simulink model "overflowtank_v000"  (R2019b)
settings: Solver=ode4  StartTime=0.0  StopTime=10000  FixedStep=1  RelTol=1e-3
libraries: simulink x5
settings Model: PauseTimes=120  Creator=engineer  LastModifiedBy=engineer

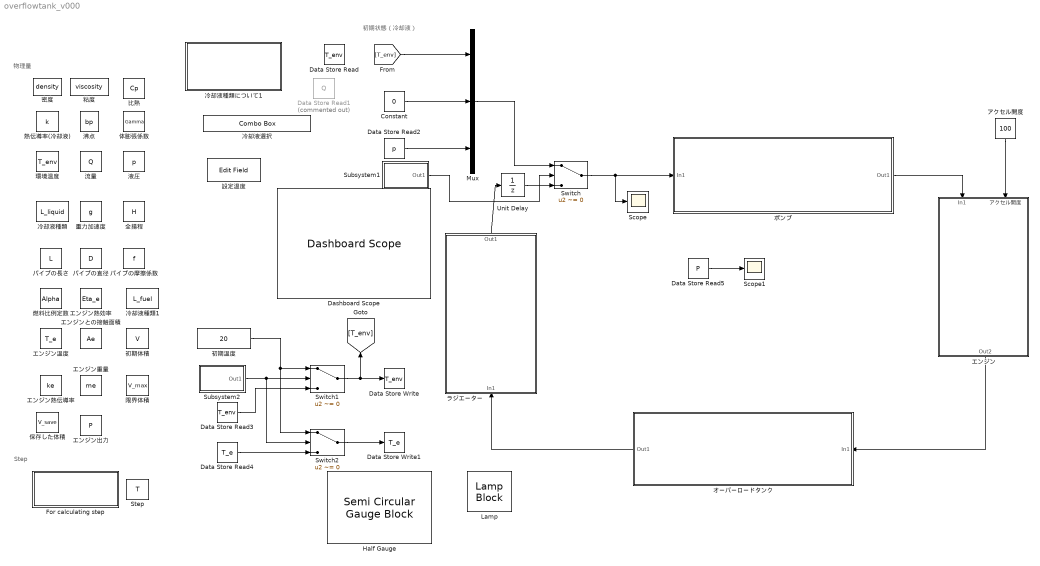
== system overflowtank_v000 ==
  note: 初期状態（冷却液）
  note: 物理量
  note: Step
  " エンジン温度" : DataStoreMemory  DataStoreName=T_e  ReadBeforeWriteMsg=warning  WriteAfterWriteMsg=warning  WriteAfterReadMsg=warning  InitialValue=25  ShowAdditionalParam=off
  " 全揚程" : DataStoreMemory  DataStoreName=H  ReadBeforeWriteMsg=warning  WriteAfterWriteMsg=warning  WriteAfterReadMsg=warning  InitialValue=2  ShowAdditionalParam=off
  " 冷却液種類" : DataStoreMemory  DataStoreName=L_liquid  ReadBeforeWriteMsg=warning  WriteAfterWriteMsg=warning  WriteAfterReadMsg=warning  ShowAdditionalParam=off  OutMin=0  OutMax=2
  " 冷却液種類1" : DataStoreMemory  DataStoreName=L_fuel  ReadBeforeWriteMsg=warning  WriteAfterWriteMsg=warning  WriteAfterReadMsg=warning  ShowAdditionalParam=off  OutMin=0  OutMax=2
  " 流量" : DataStoreMemory  DataStoreName=Q  ReadBeforeWriteMsg=warning  WriteAfterWriteMsg=warning  WriteAfterReadMsg=warning  ShowAdditionalParam=off
  " 液圧" : DataStoreMemory  DataStoreName=p  ReadBeforeWriteMsg=warning  WriteAfterWriteMsg=warning  WriteAfterReadMsg=warning  InitialValue=101  ShowAdditionalParam=off
  " 重力加速度" : DataStoreMemory  DataStoreName=g  ReadBeforeWriteMsg=warning  WriteAfterWriteMsg=warning  WriteAfterReadMsg=warning  InitialValue=10  ShowAdditionalParam=off
  Constant : Constant  Value=0
  Dashboard Scope : DashboardScope
  Data Store Read : DataStoreRead  DataStoreName=T_env
  Data Store Read1 : DataStoreRead  Commented=on  DataStoreName=Q
  Data Store Read2 : DataStoreRead  DataStoreName=p
  Data Store Read3 : DataStoreRead  DataStoreName=T_env
  Data Store Read4 : DataStoreRead  DataStoreName=T_e
  Data Store Read5 : DataStoreRead  DataStoreName=P
  Data Store Write : DataStoreWrite  DataStoreName=T_env
  Data Store Write1 : DataStoreWrite  DataStoreName=T_e
  For calculating step : Subsystem
  Half Gauge : SemiCircularGaugeBlock  ScaleMax=50
  Lamp : LampBlock
  Mux : Mux  Inputs=3
  Scope : Scope
  Scope1 : Scope
  Step : DataStoreMemory  DataStoreName=T  ReadBeforeWriteMsg=warning  WriteAfterWriteMsg=warning  WriteAfterReadMsg=warning  ShowAdditionalParam=off
  Subsystem1 : Subsystem
  Subsystem2 : Subsystem
  Switch : Switch  Criteria=u2 ~= 0
  Switch1 : Switch  Criteria=u2 ~= 0
  Switch2 : Switch  Criteria=u2 ~= 0
  Unit Delay : UnitDelay  SampleTime=-1  HasFrameUpgradeWarning=on
  アクセル開度 : Constant  Value=100
  エンジン : Subsystem
  エンジンとの接触面積 : DataStoreMemory  DataStoreName=Ae  ReadBeforeWriteMsg=warning  WriteAfterWriteMsg=warning  WriteAfterReadMsg=warning  InitialValue=0.3  ShowAdditionalParam=off
  エンジン出力 : DataStoreMemory  DataStoreName=P  ReadBeforeWriteMsg=warning  WriteAfterWriteMsg=warning  WriteAfterReadMsg=warning  ShowAdditionalParam=off
  エンジン熱伝導率 : DataStoreMemory  DataStoreName=ke  ReadBeforeWriteMsg=warning  WriteAfterWriteMsg=warning  WriteAfterReadMsg=warning  InitialValue=237  ShowAdditionalParam=off
  エンジン熱効率 : DataStoreMemory  DataStoreName=Eta_e  ReadBeforeWriteMsg=warning  WriteAfterWriteMsg=warning  WriteAfterReadMsg=warning  InitialValue=0.1  ShowAdditionalParam=off
  エンジン重量 : DataStoreMemory  DataStoreName=me  ReadBeforeWriteMsg=warning  WriteAfterWriteMsg=warning  WriteAfterReadMsg=warning  InitialValue=550  ShowAdditionalParam=off
  オーバーロードタンク : Subsystem
  パイプの摩擦係数 : DataStoreMemory  DataStoreName=f  ReadBeforeWriteMsg=warning  WriteAfterWriteMsg=warning  WriteAfterReadMsg=warning  InitialValue=0.01  ShowAdditionalParam=off
  パイプの直径 : DataStoreMemory  DataStoreName=D  ReadBeforeWriteMsg=warning  WriteAfterWriteMsg=warning  WriteAfterReadMsg=warning  InitialValue=0.04  ShowAdditionalParam=off
  パイプの長さ : DataStoreMemory  DataStoreName=L  ReadBeforeWriteMsg=warning  WriteAfterWriteMsg=warning  WriteAfterReadMsg=warning  InitialValue=7  ShowAdditionalParam=off
  ポンプ : Subsystem
  ラジエーター : Subsystem
  体膨張係数 : DataStoreMemory  DataStoreName=Gamma  ReadBeforeWriteMsg=warning  WriteAfterWriteMsg=warning  WriteAfterReadMsg=warning  InitialValue=0.00021  ShowAdditionalParam=off
  保存した体積 : DataStoreMemory  DataStoreName=V_save  InitialValue=0.001  ShowAdditionalParam=off
  冷却液種類について1 : Subsystem  VariantControl=Variant1
  冷却液選択 : ComboBox  LabelPosition=Hide  SelectedLabel=Water
      settings: Values={{'Water', 'EG30%', 'EG50%'}, [0 1 2]}
  初期体積 : DataStoreMemory  DataStoreName=V  InitialValue=0.009  ShowAdditionalParam=off
  初期温度 : Constant  Value=20
  密度 : DataStoreMemory  DataStoreName=density  ReadBeforeWriteMsg=warning  WriteAfterWriteMsg=warning  WriteAfterReadMsg=warning  InitialValue=1000  ShowAdditionalParam=off
  比熱 : DataStoreMemory  DataStoreName=Cp  ReadBeforeWriteMsg=warning  WriteAfterWriteMsg=warning  WriteAfterReadMsg=warning  InitialValue=4184  ShowAdditionalParam=off
  沸点 : DataStoreMemory  DataStoreName=bp  ReadBeforeWriteMsg=warning  WriteAfterWriteMsg=warning  WriteAfterReadMsg=warning  InitialValue=100  ShowAdditionalParam=off
  熱伝導率(冷却液) : DataStoreMemory  DataStoreName=k  ReadBeforeWriteMsg=warning  WriteAfterWriteMsg=warning  WriteAfterReadMsg=warning  InitialValue=0.606  ShowAdditionalParam=off
  燃料比例定数 : DataStoreMemory  DataStoreName=Alpha  ReadBeforeWriteMsg=warning  WriteAfterWriteMsg=warning  WriteAfterReadMsg=warning  InitialValue=0.005  ShowAdditionalParam=off
  "環境温度 " : DataStoreMemory  DataStoreName=T_env  ReadBeforeWriteMsg=warning  WriteAfterWriteMsg=warning  WriteAfterReadMsg=warning  InitialValue=25  ShowAdditionalParam=off
  粘度 : DataStoreMemory  DataStoreName=viscosity  ReadBeforeWriteMsg=warning  WriteAfterWriteMsg=warning  WriteAfterReadMsg=warning  InitialValue=0.001  ShowAdditionalParam=off
  設定温度 : EditField  LabelPosition=Hide  ShowInitialText=on  Alignment=Center
  限界体積 : DataStoreMemory  DataStoreName=V_max  InitialValue=0.009  ShowAdditionalParam=off
  wires:
  Mux/1 -> Switch/1
  [T_env] -> Mux/1
  Constant/1 -> Mux/2
  Data Store Read2/1 -> Mux/3
  Switch/1 -> ポンプ/1(In1), Scope/1
  オーバーロードタンク/1(Out1) -> ラジエーター/1(In1)
  Subsystem1/1(Out1) -> Switch/2
  Unit Delay/1 -> Switch/3
  アクセル開度/1 -> エンジン/2(アクセル開度)
  ポンプ/1(Out1) -> エンジン/1(In1)
  エンジン/1(Out2) -> オーバーロードタンク/1(In1)
  ラジエーター/1(Out1) -> Unit Delay/1
  初期温度/1 -> Switch1/1, Switch2/1
  Subsystem2/1(Out1) -> Switch2/2, Switch1/2
  Switch1/1 -> Data Store Write/1, [T_env]
  Switch2/1 -> Data Store Write1/1
  Data Store Read3/1 -> Switch1/3
  Data Store Read4/1 -> Switch2/3
  Data Store Read5/1 -> Scope1/1

== system overflowtank_v000/For calculating step ==
  Add1 : Sum  Inputs=+-
  Clock1 : Clock
  Data Store Write : DataStoreWrite  DataStoreName=T
  Unit Delay2 : UnitDelay  SampleTime=-1  HasFrameUpgradeWarning=on
  wires:
  Clock1/1 -> Add1/1, Unit Delay2/1
  Add1/1 -> Data Store Write/1
  Unit Delay2/1 -> Add1/2

== system overflowtank_v000/Subsystem1 ==
  Constant : Constant  OutDataTypeStr=boolean
  Logical Operator : Logic  Operator=NOT  AllPortsSameDT=off  OutDataTypeStr=boolean
  Logical Operator1 : Logic  AllPortsSameDT=off  OutDataTypeStr=boolean
  Unit Delay : UnitDelay  SampleTime=-1  HasFrameUpgradeWarning=on
  Out1 : Outport
  wires:
  Constant/1 -> Unit Delay/1, Logical Operator1/1
  Logical Operator/1 -> Logical Operator1/2
  Unit Delay/1 -> Logical Operator/1
  Logical Operator1/1 -> Out1/1

== system overflowtank_v000/Subsystem2 ==
  Constant : Constant  OutDataTypeStr=boolean
  Logical Operator : Logic  Operator=NOT  AllPortsSameDT=off  OutDataTypeStr=boolean
  Logical Operator1 : Logic  AllPortsSameDT=off  OutDataTypeStr=boolean
  Unit Delay : UnitDelay  SampleTime=-1  HasFrameUpgradeWarning=on
  Out1 : Outport
  wires:
  Constant/1 -> Unit Delay/1, Logical Operator1/1
  Logical Operator/1 -> Logical Operator1/2
  Unit Delay/1 -> Logical Operator/1
  Logical Operator1/1 -> Out1/1

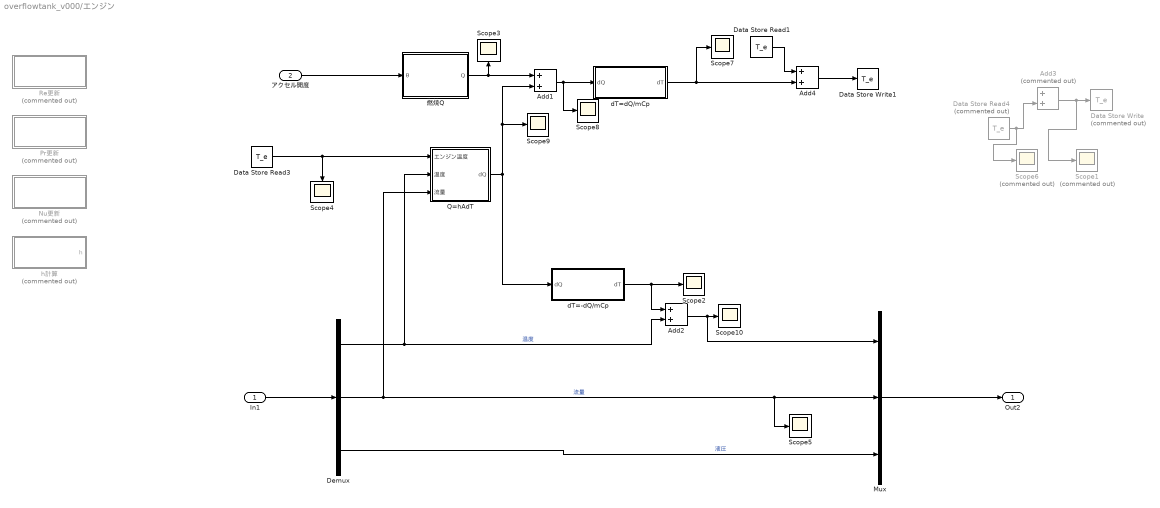
== system overflowtank_v000/エンジン ==
  In1 : Inport
  アクセル開度 : Inport  Port=2
  Add1 : Sum
  Add2 : Sum
  Add3 : Sum  Commented=on
  Add4 : Sum
  Data Store Read1 : DataStoreRead  DataStoreName=T_e
  Data Store Read3 : DataStoreRead  DataStoreName=T_e
  Data Store Read4 : DataStoreRead  Commented=on  DataStoreName=T_e
  Data Store Write : DataStoreWrite  Commented=on  DataStoreName=T_e
  Data Store Write1 : DataStoreWrite  DataStoreName=T_e
  Demux : Demux  Outputs=3
  Mux : Mux  Inputs=3
  Nu更新 : Subsystem  Commented=on
  Pr更新 : Subsystem  Commented=on
  Q=hAdT : Subsystem
  Re更新 : Subsystem  Commented=on
  Scope1 : Scope  Commented=on
  Scope{2..5,7..10} (8 alike) : Scope
  Scope6 : Scope  Commented=on
  dT=-dQ/mCp : Subsystem
  dT=dQ/mCp : Subsystem
  h計算 : Subsystem  Commented=on
  "燃焼Q " : Subsystem
  Out2 : Outport
  wires:
  In1/1 -> Demux/1
  Mux/1 -> Out2/1
  アクセル開度/1 -> "燃焼Q "/1(θ)
  Data Store Read3/1 -> Scope4/1, Q=hAdT/1(エンジン温度)
  "燃焼Q "/1(Q) -> Scope3/1, Add1/1
  Demux/1 -> Add2/2, Q=hAdT/2(温度)  "温度"
  Demux/2 -> Mux/2, Scope5/1, Q=hAdT/3(流量)  "流量"
  Demux/3 -> Mux/3  "液圧"
  dT=-dQ/mCp/1(dT) -> Add2/1, Scope2/1
  Add1/1 -> dT=dQ/mCp/1(dQ), Scope8/1
  dT=dQ/mCp/1(dT) -> Add4/2, Scope7/1
  Data Store Read4/1 -> Scope6/1, Add3/2
  Add3/1 -> Scope1/1, Data Store Write/1
  Data Store Read1/1 -> Add4/1
  Add4/1 -> Data Store Write1/1
  Add2/1 -> Mux/1, Scope10/1
  Q=hAdT/1(dQ) -> Add1/2, Scope9/1, dT=-dQ/mCp/1(dQ)

== system overflowtank_v000/オーバーロードタンク ==
  In1 : Inport
  Data Store Read : DataStoreRead  DataStoreName=V_save
  Demux : Demux  Outputs=3
  Mux : Mux  Inputs=3
  Scope : Scope
  Scope1 : Scope
  V=V0(1+γdT) : Subsystem
  オーバーフロータンク制御 : Subsystem
  Out1 : Outport
  wires:
  In1/1 -> Demux/1
  Mux/1 -> Out1/1
  Demux/1 -> V=V0(1+γdT)/1(温度), Mux/1  "温度"
  Demux/2 -> Mux/2  "流量"
  Demux/3 -> Mux/3  "液圧"
  V=V0(1+γdT)/1(実体積) -> オーバーフロータンク制御/1(実体積), Scope/1
  Data Store Read/1 -> Scope1/1

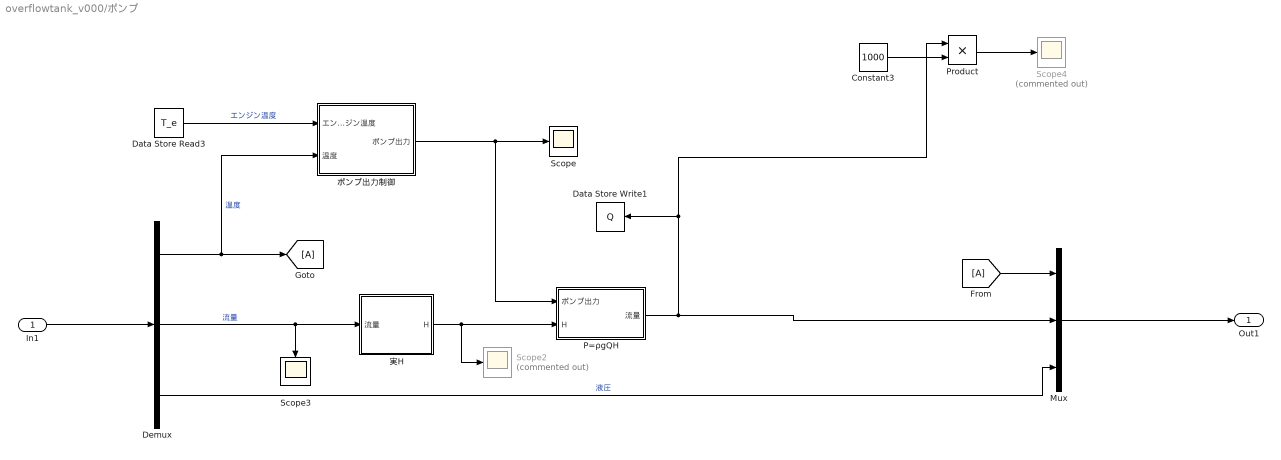
== system overflowtank_v000/ポンプ ==
  In1 : Inport
  Constant3 : Constant  Value=1000
  Data Store Read3 : DataStoreRead  DataStoreName=T_e
  Data Store Write1 : DataStoreWrite  DataStoreName=Q
  Demux : Demux  Outputs=3
  Mux : Mux  Inputs=3
  P=ρgQH : Subsystem
  Product : Product
  Scope : Scope
  Scope2 : Scope  Commented=on
  Scope3 : Scope
  Scope4 : Scope  Commented=on
  ポンプ出力制御 : Subsystem
  実H : Subsystem
  Out1 : Outport
  wires:
  In1/1 -> Demux/1
  Demux/3 -> Mux/3  "液圧"
  Demux/1 -> ポンプ出力制御/2(温度), [A]  "温度"
  P=ρgQH/1(流量) -> Product/1, Data Store Write1/1, Mux/2
  Mux/1 -> Out1/1
  Demux/2 -> 実H/1(流量), Scope3/1  "流量"
  実H/1(H) -> P=ρgQH/2(H), Scope2/1
  [A] -> Mux/1
  Constant3/1 -> Product/2
  Product/1 -> Scope4/1
  ポンプ出力制御/1(ポンプ出力) -> P=ρgQH/1(ポンプ出力), Scope/1
  Data Store Read3/1 -> ポンプ出力制御/1(エンジン温度)  "エンジン温度"

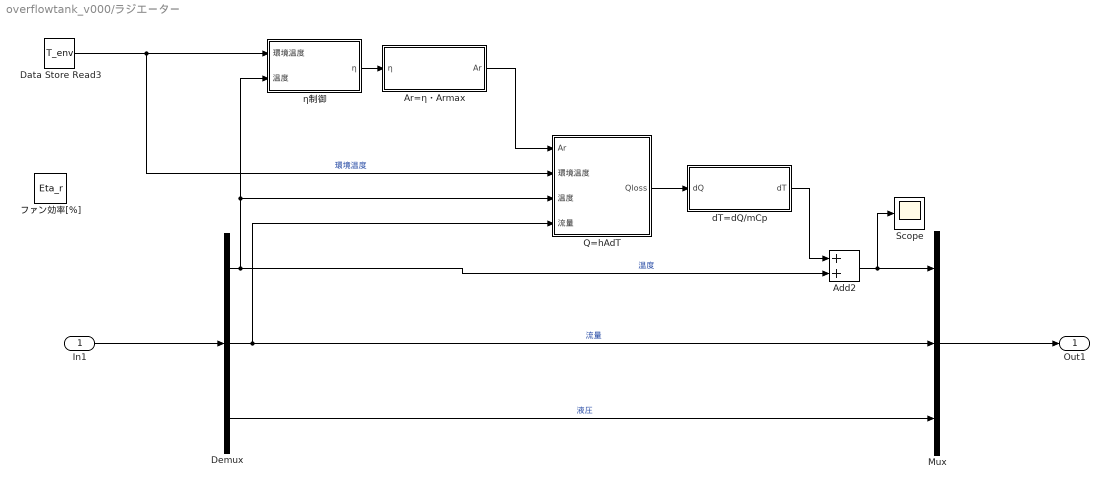
== system overflowtank_v000/ラジエーター ==
  In1 : Inport
  Add2 : Sum
  Ar=η・Armax : Subsystem
  Data Store Read3 : DataStoreRead  DataStoreName=T_env
  Demux : Demux  Outputs=3
  Mux : Mux  Inputs=3
  Q=hAdT : Subsystem
  Scope : Scope
  dT=dQ/mCp : Subsystem
  η制御 : Subsystem
  ファン効率[%] : DataStoreMemory  DataStoreName=Eta_r  ReadBeforeWriteMsg=warning  WriteAfterWriteMsg=warning  WriteAfterReadMsg=warning  InitialValue=0.75  ShowAdditionalParam=off  OutMin=0  OutMax=100
  Out1 : Outport
  wires:
  Mux/1 -> Out1/1
  In1/1 -> Demux/1
  Demux/2 -> Q=hAdT/4(流量), Mux/2  "流量"
  Demux/3 -> Mux/3  "液圧"
  Demux/1 -> Q=hAdT/3(温度), η制御/2(温度), Add2/2  "温度"
  dT=dQ/mCp/1(dT) -> Add2/1
  Add2/1 -> Mux/1, Scope/1
  Data Store Read3/1 -> Q=hAdT/2(環境温度), η制御/1(環境温度)  "環境温度"
  η制御/1(η) -> Ar=η・Armax/1(η)
  Ar=η・Armax/1(Ar) -> Q=hAdT/1("Ar ")
  Q=hAdT/1(Qloss) -> dT=dQ/mCp/1(dQ)

== system overflowtank_v000/冷却液種類について1 ==
  AND : Logic  IconShape=distinctive  AllPortsSameDT=off  OutDataTypeStr=boolean
  AND1 : Logic  IconShape=distinctive  AllPortsSameDT=off  OutDataTypeStr=boolean
  AND2 : Logic  IconShape=distinctive  AllPortsSameDT=off  OutDataTypeStr=boolean
  Compare To Constant : simulink/Logic and Bit Operations/Compare To Constant  relop===  const=0  OutDataTypeStr=boolean
  Compare To Constant1 : simulink/Logic and Bit Operations/Compare To Constant  relop===  const=1  OutDataTypeStr=boolean
  Compare To Constant2 : simulink/Logic and Bit Operations/Compare To Constant  relop===  const=2  OutDataTypeStr=boolean
  Data Store Read3 : DataStoreRead  DataStoreName=L_liquid
  Enabled Subsystem : Subsystem  TreatAsAtomicUnit=on
  Enabled Subsystem1 : Subsystem  TreatAsAtomicUnit=on
  Enabled Subsystem3 : Subsystem  TreatAsAtomicUnit=on
  Subsystem1 : Subsystem
  wires:
  Compare To Constant/1 -> AND/1  "水"
  Data Store Read3/1 -> Compare To Constant2/1, Compare To Constant1/1, Compare To Constant/1
  Compare To Constant1/1 -> AND1/1  "EG(30%)"
  Compare To Constant2/1 -> AND2/1  "EG(50%)"
  AND/1 -> Enabled Subsystem/Enable
  Subsystem1/1(Out1) -> AND2/2, AND1/2, AND/2
  AND1/1 -> Enabled Subsystem3/Enable
  AND2/1 -> Enabled Subsystem1/Enable

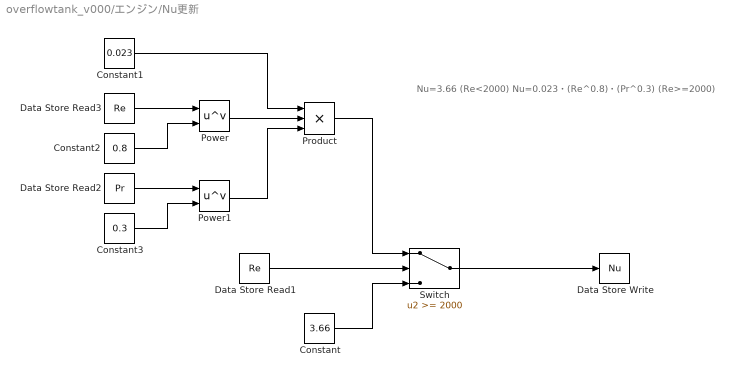
== system overflowtank_v000/エンジン/Nu更新 ==
  note: Nu=3.66 (Re<2000)
      | Nu=0.023・(Re^0.8)・(Pr^0.3) (Re>=2000)
  Constant : Constant  Value=3.66
  Constant1 : Constant  Value=0.023
  Constant2 : Constant  Value=0.8
  Constant3 : Constant  Value=0.3
  Data Store Read1 : DataStoreRead  DataStoreName=Re
  Data Store Read2 : DataStoreRead  DataStoreName=Pr
  Data Store Read3 : DataStoreRead  DataStoreName=Re
  Data Store Write : DataStoreWrite  DataStoreName=Nu
  Power : Math  Operator=pow  SignedPower=off  SaturateOnIntegerOverflow=on
  Power1 : Math  Operator=pow  SignedPower=off  SaturateOnIntegerOverflow=on
  Product : Product  Inputs=3
  Switch : Switch  Threshold=2000
  wires:
  Constant/1 -> Switch/3
  Switch/1 -> Data Store Write/1
  Data Store Read1/1 -> Switch/2
  Data Store Read3/1 -> Power/1
  Constant2/1 -> Power/2
  Data Store Read2/1 -> Power1/1
  Constant3/1 -> Power1/2
  Constant1/1 -> Product/1
  Power/1 -> Product/2
  Power1/1 -> Product/3
  Product/1 -> Switch/1

== system overflowtank_v000/エンジン/Pr更新 ==
  note: Pr=μ・Cp/k
  Data Store Read : DataStoreRead  DataStoreName=Cp
  Data Store Read2 : DataStoreRead  DataStoreName=viscosity
  Data Store Read3 : DataStoreRead  DataStoreName=ke
  Data Store Write : DataStoreWrite  DataStoreName=Pr
  Divide : Product  Inputs=*/
  Product : Product
  wires:
  Data Store Read2/1 -> Product/2
  Data Store Read/1 -> Product/1
  Product/1 -> Divide/1
  Data Store Read3/1 -> Divide/2
  Divide/1 -> Data Store Write/1

== system overflowtank_v000/エンジン/Q=hAdT ==
  エンジン温度 : Inport
  温度 : Inport  Port=2
  流量 : Inport  Port=3
  Add : Sum  Inputs=+-
  Data Store Read2 : DataStoreRead  DataStoreName=Ae
  Product : Product  Inputs=3
  "h計算 " : Subsystem
  dQ : Outport
  wires:
  エンジン温度/1 -> Add/2
  Add/1 -> Product/1
  "h計算 "/1(h) -> Product/3
  Product/1 -> dQ/1  "Qloss"
  Data Store Read2/1 -> Product/2
  流量/1 -> "h計算 "/1(流量Q)
  温度/1 -> Add/1

== system overflowtank_v000/エンジン/Re更新 ==
  note: Re=4ρQ/ΠμD
  Constant : Constant  Value=4
  Constant1 : Constant  Value=pi
  Data Store Read : DataStoreRead  DataStoreName=density
  Data Store Read1 : DataStoreRead  DataStoreName=Q
  Data Store Read2 : DataStoreRead  DataStoreName=viscosity
  Data Store Read3 : DataStoreRead  DataStoreName=D
  Data Store Write : DataStoreWrite  DataStoreName=Re
  Divide : Product  Inputs=*/
  Product : Product  Inputs=3
  Product1 : Product  Inputs=3
  wires:
  Constant/1 -> Product/1
  Data Store Read/1 -> Product/2
  Data Store Read1/1 -> Product/3
  Product/1 -> Divide/1
  Data Store Read2/1 -> Product1/2
  Constant1/1 -> Product1/1
  Data Store Read3/1 -> Product1/3
  Product1/1 -> Divide/2
  Divide/1 -> Data Store Write/1

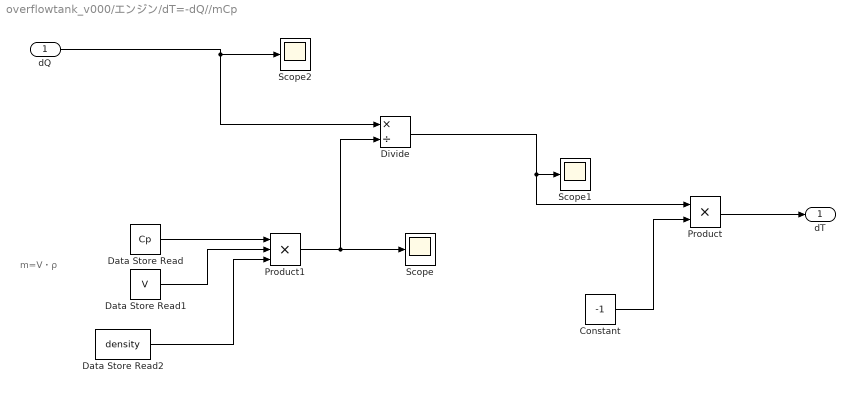
== system overflowtank_v000/エンジン/dT=-dQ//mCp ==
  note: m=V・ρ
  dQ : Inport
  Constant : Constant  Value=-1
  Data Store Read : DataStoreRead  DataStoreName=Cp
  Data Store Read1 : DataStoreRead  DataStoreName=V
  Data Store Read2 : DataStoreRead  DataStoreName=density
  Divide : Product  Inputs=*/
  Product : Product
  Product1 : Product  Inputs=3
  Scope : Scope
  Scope1 : Scope
  Scope2 : Scope
  dT : Outport
  wires:
  dQ/1 -> Scope2/1, Divide/1
  Data Store Read/1 -> Product1/1
  Data Store Read1/1 -> Product1/2
  Data Store Read2/1 -> Product1/3
  Product1/1 -> Divide/2, Scope/1
  Divide/1 -> Product/1, Scope1/1
  Constant/1 -> Product/2
  Product/1 -> dT/1

== system overflowtank_v000/エンジン/dT=dQ//mCp ==
  dQ : Inport
  "Cp " : Constant  Value=880
  Data Store Read1 : DataStoreRead  DataStoreName=me
  Divide : Product  Inputs=*/
  Product1 : Product
  dT : Outport
  wires:
  dQ/1 -> Divide/1
  "Cp "/1 -> Product1/1
  Data Store Read1/1 -> Product1/2
  Product1/1 -> Divide/2
  Divide/1 -> dT/1

== system overflowtank_v000/エンジン/h計算 ==
  note: h=(k/D)・Nu(Re,Pr)
  Data Store Read : DataStoreRead  DataStoreName=Nu
  Data Store Read1 : DataStoreRead  DataStoreName=D
  Data Store Read3 : DataStoreRead  DataStoreName=ke
  Divide : Product  Inputs=*/
  Product : Product
  h : Outport
  wires:
  Data Store Read3/1 -> Divide/1
  Divide/1 -> Product/1
  Data Store Read1/1 -> Divide/2
  Product/1 -> h/1
  Data Store Read/1 -> Product/2

== system overflowtank_v000/エンジン/燃焼Q  ==
  note: Q=mf・LHV・ η
  θ : Inport
  Data Store Read3 : DataStoreRead  DataStoreName=Eta_e
  Product : Product  Inputs=3
  Subsystem : Subsystem
  mf=αθ : Subsystem
  Q : Outport
  wires:
  mf=αθ/1(mf) -> Product/1
  Data Store Read3/1 -> Product/2
  Product/1 -> Q/1  "Q"
  Subsystem/1("LHV ") -> Product/3
  θ/1 -> mf=αθ/1(θ)

== system overflowtank_v000/オーバーロードタンク/V=V0(1+γdT) ==
  温度 : Inport
  Add : Sum
  Data Store Read1 : DataStoreRead  DataStoreName=Gamma
  Data Store Read2 : DataStoreRead  DataStoreName=T_env
  Data Store Read3 : DataStoreRead  DataStoreName=V
  Data Store Read4 : DataStoreRead  DataStoreName=V
  Plus1 : Sum  Inputs=-+
  Product : Product  Inputs=3
  実体積 : Outport
  wires:
  Data Store Read1/1 -> Product/2
  Data Store Read3/1 -> Product/1
  温度/1 -> Plus1/2
  Plus1/1 -> Product/3
  Data Store Read2/1 -> Plus1/1
  Product/1 -> Add/1
  Data Store Read4/1 -> Add/2
  Add/1 -> 実体積/1

== system overflowtank_v000/オーバーロードタンク/オーバーフロータンク制御 ==
  note: 体積の差
  note: 取る
  実体積 : Inport
  Add : Sum
  Constant : Constant  Value=0
  Data Store Read : DataStoreRead  DataStoreName=V_save
  Data Store Read4 : DataStoreRead  DataStoreName=V_max
  Data Store Write : DataStoreWrite  DataStoreName=V_save
  Max : MinMax  Function=max  Inputs=2
  Plus1 : Sum  Inputs=+-
  Scope1 : Scope
  Switch : Switch  Criteria=u2 > Threshold
  wires:
  Constant/1 -> Max/2
  Add/1 -> Max/1
  Switch/1 -> Scope1/1, Data Store Write/1
  Data Store Read4/1 -> Plus1/2
  Data Store Read/1 -> Add/2
  Plus1/1 -> Switch/1, Switch/2, Add/1  "保存"
  Max/1 -> Switch/3
  実体積/1 -> Plus1/1

== system overflowtank_v000/ポンプ/P=ρgQH ==
  note: P=ρgQH
  ポンプ出力 : Inport
  H : Inport  Port=2
  Data Store Read3 : DataStoreRead  DataStoreName=density
  Data Store Read4 : DataStoreRead  DataStoreName=g
  Divide : Product  Inputs=*/
  Product : Product  Inputs=3
  Scope : Scope
  Scope1 : Scope
  流量 : Outport
  wires:
  H/1 -> Product/3
  Data Store Read3/1 -> Product/1
  ポンプ出力/1 -> Divide/1
  Data Store Read4/1 -> Product/2
  Product/1 -> Scope/1, Divide/2
  Divide/1 -> Scope1/1, 流量/1  "流量"

== system overflowtank_v000/ポンプ/ポンプ出力制御 ==
  note: 温度の差について
  エンジン温度 : Inport
  温度 : Inport  Port=2
  Constant : Constant  Value=5
  Data Store Write : DataStoreWrite  DataStoreName=P
  Plus : Sum  Inputs=+-
  Relational Operator : RelationalOperator  Operator=>  OutDataTypeStr=boolean  RndMeth=Simplest
  Switch : Switch  Criteria=u2 ~= 0
  ポンプ出力DOWN : Subsystem
  ポンプ出力UP : Subsystem
  ポンプ出力 : Outport
  wires:
  ポンプ出力UP/1(Out1) -> Switch/1
  エンジン温度/1 -> Plus/1
  Constant/1 -> Plus/2
  ポンプ出力DOWN/1(Out1) -> Switch/3
  Switch/1 -> Data Store Write/1, ポンプ出力/1
  Plus/1 -> Relational Operator/1
  Relational Operator/1 -> Switch/2
  温度/1 -> Relational Operator/2

== system overflowtank_v000/ポンプ/実H ==
  note: 液圧の差を省略する
  流量 : Inport
  Scope : Scope
  Scope1 : Scope
  hf=(fLv^2)/(2gD) : Subsystem
  v=Q/A : Subsystem
  ベルヌーイの定理 : Subsystem
  H : Outport
  wires:
  流量/1 -> Scope1/1, v=Q/A/1(Q)
  hf=(fLv^2)/(2gD)/1(hf) -> ベルヌーイの定理/1(hf)
  v=Q/A/1(v) -> ベルヌーイの定理/2(v), hf=(fLv^2)/(2gD)/1(v)
  ベルヌーイの定理/1(H) -> Scope/1, H/1

== system overflowtank_v000/ラジエーター/Ar=η・Armax ==
  η : Inport
  Product : Product
  冷却ファンの最大表面積 : Constant  Value=0.2
  Ar : Outport
  wires:
  η/1 -> Product/1
  Product/1 -> Ar/1
  冷却ファンの最大表面積/1 -> Product/2

== system overflowtank_v000/ラジエーター/Q=hAdT ==
  "Ar " : Inport
  環境温度 : Inport  Port=2
  温度 : Inport  Port=3
  流量 : Inport  Port=4
  Add : Sum  Inputs=+-
  Product : Product  Inputs=3
  h計算 : Subsystem
  Qloss : Outport
  wires:
  h計算/1(h) -> Product/3
  Add/1 -> Product/2
  環境温度/1 -> Add/1
  "Ar "/1 -> Product/1
  Product/1 -> Qloss/1  "Qloss"
  流量/1 -> h計算/1(流量Q)
  温度/1 -> Add/2

== system overflowtank_v000/ラジエーター/dT=dQ//mCp ==
  note: m=V・ρ
  dQ : Inport
  Data Store Read : DataStoreRead  DataStoreName=Cp
  Data Store Read1 : DataStoreRead  DataStoreName=V
  Data Store Read2 : DataStoreRead  DataStoreName=density
  Divide : Product  Inputs=*/
  Product1 : Product  Inputs=3
  Scope : Scope
  Scope1 : Scope
  Scope2 : Scope
  dT : Outport
  wires:
  dQ/1 -> Scope2/1, Divide/1
  Data Store Read/1 -> Product1/1
  Data Store Read1/1 -> Product1/2
  Data Store Read2/1 -> Product1/3
  Product1/1 -> Divide/2, Scope/1
  Divide/1 -> dT/1, Scope1/1

== system overflowtank_v000/ラジエーター/η制御 ==
  note: 温度の差について
  環境温度 : Inport
  温度 : Inport  Port=2
  Constant : Constant  Value=5
  Data Store Write : DataStoreWrite  DataStoreName=Eta_r
  Eta_rDOWN : Subsystem
  "Eta_rUP " : Subsystem
  Plus : Sum
  Relational Operator : RelationalOperator  Operator=<  OutDataTypeStr=boolean  RndMeth=Simplest
  Scope1 : Scope
  Switch : Switch  Criteria=u2 ~= 0
  η : Outport
  wires:
  Relational Operator/1 -> Switch/2
  Plus/1 -> Relational Operator/1
  Switch/1 -> η/1, Data Store Write/1, Scope1/1
  Eta_rDOWN/1(η) -> Switch/3
  Constant/1 -> Plus/1
  温度/1 -> Relational Operator/2
  "Eta_rUP "/1(η) -> Switch/1
  環境温度/1 -> Plus/2

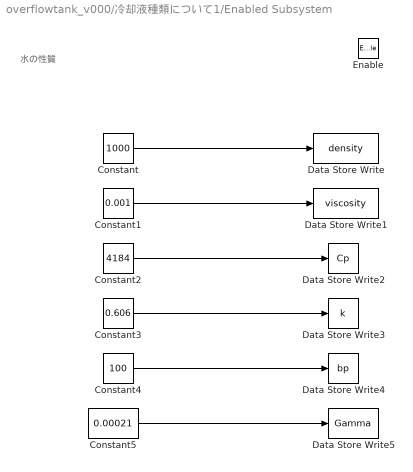
== system overflowtank_v000/冷却液種類について1/Enabled Subsystem ==
  note: 水の性質
  Enable : EnablePort
  Constant : Constant  Value=1000
  Constant1 : Constant  Value=0.001
  Constant2 : Constant  Value=4184
  Constant3 : Constant  Value=0.606
  Constant4 : Constant  Value=100
  Constant5 : Constant  Value=0.00021
  Data Store Write : DataStoreWrite  DataStoreName=density
  Data Store Write1 : DataStoreWrite  DataStoreName=viscosity
  Data Store Write2 : DataStoreWrite  DataStoreName=Cp
  Data Store Write3 : DataStoreWrite  DataStoreName=k
  Data Store Write4 : DataStoreWrite  DataStoreName=bp
  Data Store Write5 : DataStoreWrite  DataStoreName=Gamma
  wires:
  Constant/1 -> Data Store Write/1
  Constant1/1 -> Data Store Write1/1
  Constant2/1 -> Data Store Write2/1
  Constant3/1 -> Data Store Write3/1
  Constant4/1 -> Data Store Write4/1
  Constant5/1 -> Data Store Write5/1

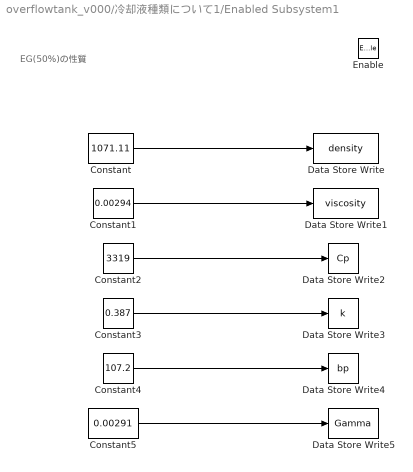
== system overflowtank_v000/冷却液種類について1/Enabled Subsystem1 ==
  note: EG(50%)の性質
  Enable : EnablePort
  Constant : Constant  Value=1071.11
  Constant1 : Constant  Value=0.00294
  Constant2 : Constant  Value=3319
  Constant3 : Constant  Value=0.387
  Constant4 : Constant  Value=107.2
  Constant5 : Constant  Value=0.00291
  Data Store Write : DataStoreWrite  DataStoreName=density
  Data Store Write1 : DataStoreWrite  DataStoreName=viscosity
  Data Store Write2 : DataStoreWrite  DataStoreName=Cp
  Data Store Write3 : DataStoreWrite  DataStoreName=k
  Data Store Write4 : DataStoreWrite  DataStoreName=bp
  Data Store Write5 : DataStoreWrite  DataStoreName=Gamma
  wires:
  Constant/1 -> Data Store Write/1
  Constant1/1 -> Data Store Write1/1
  Constant2/1 -> Data Store Write2/1
  Constant3/1 -> Data Store Write3/1
  Constant4/1 -> Data Store Write4/1
  Constant5/1 -> Data Store Write5/1

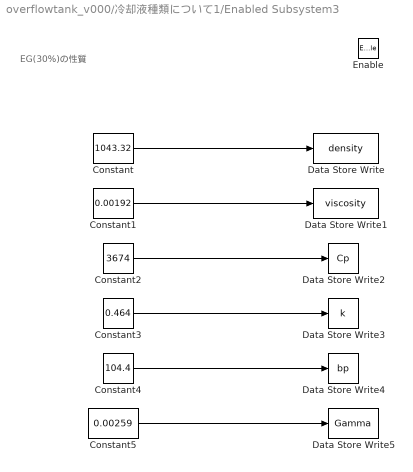
== system overflowtank_v000/冷却液種類について1/Enabled Subsystem3 ==
  note: EG(30%)の性質
  Enable : EnablePort
  Constant : Constant  Value=1043.32
  Constant1 : Constant  Value=0.00192
  Constant2 : Constant  Value=3674
  Constant3 : Constant  Value=0.464
  Constant4 : Constant  Value=104.4
  Constant5 : Constant  Value=0.00259
  Data Store Write : DataStoreWrite  DataStoreName=density
  Data Store Write1 : DataStoreWrite  DataStoreName=viscosity
  Data Store Write2 : DataStoreWrite  DataStoreName=Cp
  Data Store Write3 : DataStoreWrite  DataStoreName=k
  Data Store Write4 : DataStoreWrite  DataStoreName=bp
  Data Store Write5 : DataStoreWrite  DataStoreName=Gamma
  wires:
  Constant/1 -> Data Store Write/1
  Constant1/1 -> Data Store Write1/1
  Constant2/1 -> Data Store Write2/1
  Constant3/1 -> Data Store Write3/1
  Constant4/1 -> Data Store Write4/1
  Constant5/1 -> Data Store Write5/1

== system overflowtank_v000/冷却液種類について1/Subsystem1 ==
  Constant : Constant  OutDataTypeStr=boolean
  Logical Operator : Logic  Operator=NOT  AllPortsSameDT=off  OutDataTypeStr=boolean
  Logical Operator1 : Logic  AllPortsSameDT=off  OutDataTypeStr=boolean
  Unit Delay : UnitDelay  SampleTime=-1  HasFrameUpgradeWarning=on
  Out1 : Outport
  wires:
  Constant/1 -> Unit Delay/1, Logical Operator1/1
  Logical Operator/1 -> Logical Operator1/2
  Unit Delay/1 -> Logical Operator/1
  Logical Operator1/1 -> Out1/1

== system overflowtank_v000/エンジン/Q=hAdT/h計算  ==
  note: h=(k/D)・Nu(Re,Pr)
  流量Q : Inport
  Data Store Read1 : DataStoreRead  DataStoreName=D
  Data Store Read3 : DataStoreRead  DataStoreName=k
  Divide : Product  Inputs=*/
  Nu更新 : Subsystem
  Product : Product
  h : Outport
  wires:
  Data Store Read3/1 -> Divide/1
  Divide/1 -> Product/1
  Data Store Read1/1 -> Divide/2
  Product/1 -> h/1
  Nu更新/1(Nu) -> Product/2
  流量Q/1 -> Nu更新/1(流量Q)

== system overflowtank_v000/エンジン/燃焼Q /Subsystem ==
  Compare To Constant : simulink/Logic and Bit Operations/Compare To Constant  relop===  const=0  OutDataTypeStr=boolean
  Compare To Constant1 : simulink/Logic and Bit Operations/Compare To Constant  relop===  const=1  OutDataTypeStr=boolean
  Constant : Constant  Value=45000000
  Constant1 : Constant  Value=47000000
  Constant2 : Constant  Value=47000000
  Data Store Read3 : DataStoreRead  DataStoreName=L_fuel
  Switch : Switch  Criteria=u2 ~= 0
  Switch1 : Switch  Criteria=u2 ~= 0
  "LHV " : Outport
  wires:
  Compare To Constant1/1 -> Switch1/2  "アルミニウム"
  Data Store Read3/1 -> Compare To Constant1/1, Compare To Constant/1
  Compare To Constant/1 -> Switch/2  "ガソリン"
  Switch/1 -> "LHV "/1
  Constant1/1 -> Switch/1
  Switch1/1 -> Switch/3
  Constant/1 -> Switch1/1
  Constant2/1 -> Switch1/3

== system overflowtank_v000/エンジン/燃焼Q /mf=αθ ==
  θ : Inport
  Constant1 : Constant  Value=0.02
  Data Store Read3 : DataStoreRead  DataStoreName=Alpha
  Product : Product  Inputs=3
  mf : Outport
  wires:
  Product/1 -> mf/1
  Data Store Read3/1 -> Product/2
  Constant1/1 -> Product/3
  θ/1 -> Product/1

== system overflowtank_v000/ポンプ/ポンプ出力制御/ポンプ出力DOWN ==
  Add : Sum  Inputs=+-
  Constant1 : Constant
  Constant2 : Constant  Value=0
  Data Store Read1 : DataStoreRead  DataStoreName=P
  Max : MinMax  Function=max  Inputs=2
  Out1 : Outport
  wires:
  Constant2/1 -> Max/2
  Add/1 -> Max/1
  Constant1/1 -> Add/2
  Data Store Read1/1 -> Add/1
  Max/1 -> Out1/1

== system overflowtank_v000/ポンプ/ポンプ出力制御/ポンプ出力UP ==
  Add : Sum
  Constant1 : Constant
  Constant2 : Constant  Value=45
  Data Store Read1 : DataStoreRead  DataStoreName=P
  Max : MinMax  Inputs=2
  Out1 : Outport
  wires:
  Constant2/1 -> Max/2
  Add/1 -> Max/1
  Constant1/1 -> Add/2
  Data Store Read1/1 -> Add/1
  Max/1 -> Out1/1

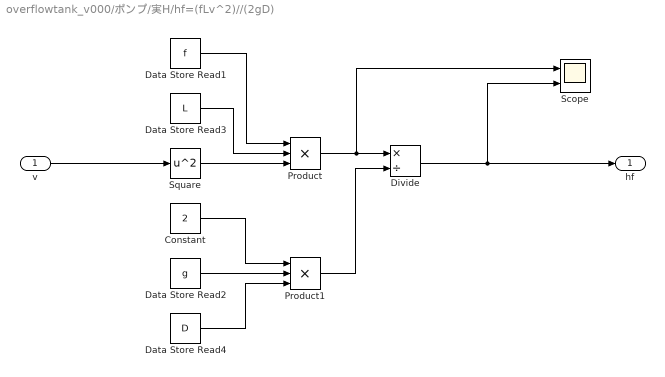
== system overflowtank_v000/ポンプ/実H/hf=(fLv^2)//(2gD) ==
  v : Inport
  Constant : Constant  Value=2
  Data Store Read1 : DataStoreRead  DataStoreName=f
  Data Store Read2 : DataStoreRead  DataStoreName=g
  Data Store Read3 : DataStoreRead  DataStoreName=L
  Data Store Read4 : DataStoreRead  DataStoreName=D
  Divide : Product  Inputs=*/
  Product : Product  Inputs=3
  Product1 : Product  Inputs=3
  Scope : Scope  NumInputPorts=2
  Square : Math  Operator=square  SignedPower=off  SaturateOnIntegerOverflow=on
  hf : Outport
  wires:
  v/1 -> Square/1
  Square/1 -> Product/3
  Data Store Read3/1 -> Product/2
  Data Store Read1/1 -> Product/1
  Product/1 -> Scope/1, Divide/1
  Constant/1 -> Product1/1
  Data Store Read2/1 -> Product1/2
  Data Store Read4/1 -> Product1/3
  Product1/1 -> Divide/2
  Divide/1 -> Scope/2, hf/1

== system overflowtank_v000/ポンプ/実H/v=Q//A ==
  Q : Inport
  A=pi*(D/2)^2 : Subsystem
  Divide1 : Product  Inputs=*/
  v : Outport
  wires:
  Q/1 -> Divide1/1
  Divide1/1 -> v/1
  A=pi*(D/2)^2/1(A) -> Divide1/2

== system overflowtank_v000/ポンプ/実H/ベルヌーイの定理 ==
  hf : Inport
  v : Inport  Port=2
  Data Store Read2 : DataStoreRead  DataStoreName=H
  Subtract : Sum  Inputs=+-
  Subtract1 : Sum  Inputs=+-
  速度ヘッド : Subsystem
  H : Outport
  wires:
  Data Store Read2/1 -> Subtract/1
  Subtract/1 -> Subtract1/1
  v/1 -> 速度ヘッド/1(v)
  速度ヘッド/1(速度ヘッド) -> Subtract1/2
  hf/1 -> Subtract/2
  Subtract1/1 -> H/1

== system overflowtank_v000/ラジエーター/Q=hAdT/h計算 ==
  note: h=(k/D)・Nu(Re,Pr)
  流量Q : Inport
  Data Store Read1 : DataStoreRead  DataStoreName=D
  Data Store Read3 : DataStoreRead  DataStoreName=k
  Divide : Product  Inputs=*/
  Nu更新 : Subsystem
  Product : Product
  h : Outport
  wires:
  Data Store Read3/1 -> Divide/1
  Divide/1 -> Product/1
  Data Store Read1/1 -> Divide/2
  Product/1 -> h/1
  Nu更新/1(Nu) -> Product/2
  流量Q/1 -> Nu更新/1(流量Q)

== system overflowtank_v000/ラジエーター/η制御/Eta_rDOWN ==
  Add1 : Sum  Inputs=+-
  Constant1 : Constant  Value=0.0002
  Constant2 : Constant  Value=0
  Data Store Read1 : DataStoreRead  DataStoreName=Eta_r
  Max : MinMax  Function=max  Inputs=2
  η : Outport
  wires:
  Constant2/1 -> Max/2
  Add1/1 -> Max/1
  Data Store Read1/1 -> Add1/1
  Constant1/1 -> Add1/2
  Max/1 -> η/1

== system overflowtank_v000/ラジエーター/η制御/Eta_rUP  ==
  Add1 : Sum
  Constant1 : Constant  Value=0.0002
  Constant2 : Constant
  Data Store Read1 : DataStoreRead  DataStoreName=Eta_r
  Max : MinMax  Inputs=2
  η : Outport
  wires:
  Constant2/1 -> Max/2
  Add1/1 -> Max/1
  Data Store Read1/1 -> Add1/1
  Constant1/1 -> Add1/2
  Max/1 -> η/1

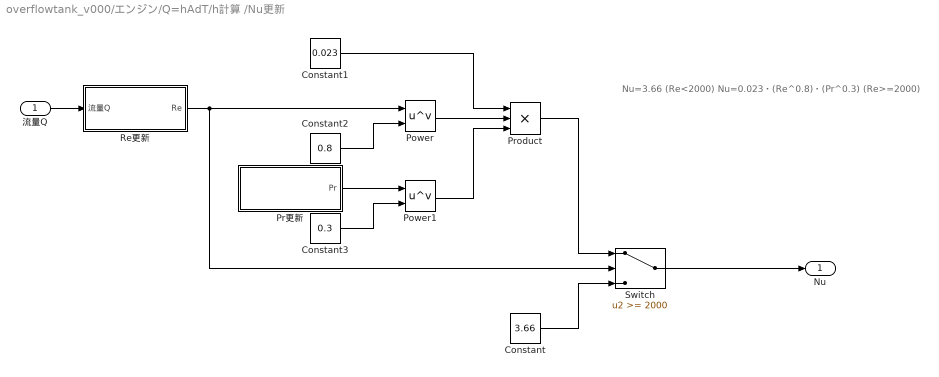
== system overflowtank_v000/エンジン/Q=hAdT/h計算 /Nu更新 ==
  note: Nu=3.66 (Re<2000)
      | Nu=0.023・(Re^0.8)・(Pr^0.3) (Re>=2000)
  流量Q : Inport
  Constant : Constant  Value=3.66
  Constant1 : Constant  Value=0.023
  Constant2 : Constant  Value=0.8
  Constant3 : Constant  Value=0.3
  Power : Math  Operator=pow  SignedPower=off  SaturateOnIntegerOverflow=on
  Power1 : Math  Operator=pow  SignedPower=off  SaturateOnIntegerOverflow=on
  Product : Product  Inputs=3
  Pr更新 : Subsystem
  Re更新 : Subsystem
  Switch : Switch  Threshold=2000
  Nu : Outport
  wires:
  Constant/1 -> Switch/3
  Switch/1 -> Nu/1
  Re更新/1(Re) -> Switch/2, Power/1
  Constant2/1 -> Power/2
  Pr更新/1(Pr) -> Power1/1
  Constant3/1 -> Power1/2
  Constant1/1 -> Product/1
  Power/1 -> Product/2
  Power1/1 -> Product/3
  Product/1 -> Switch/1
  流量Q/1 -> Re更新/1(流量Q)

== system overflowtank_v000/ポンプ/実H/v=Q//A/A=pi*(D//2)^2 ==
  Constant : Constant  Value=2
  Data Store Read3 : DataStoreRead  DataStoreName=D
  Divide : Product  Inputs=*/
  Pi : Constant  Value=pi  OutDataTypeStr=Inherit: Inherit via back propagation
  Product : Product
  Square : Math  Operator=square  SignedPower=off  SaturateOnIntegerOverflow=on
  A : Outport
  wires:
  Constant/1 -> Divide/2
  Divide/1 -> Square/1
  Data Store Read3/1 -> Divide/1
  Product/1 -> A/1
  Pi/1 -> Product/2
  Square/1 -> Product/1

== system overflowtank_v000/ポンプ/実H/ベルヌーイの定理/速度ヘッド ==
  v : Inport
  Constant : Constant  Value=2
  Data Store Read1 : DataStoreRead  DataStoreName=g
  Divide : Product  Inputs=*/
  Product : Product
  Square : Math  Operator=square  SignedPower=off  SaturateOnIntegerOverflow=on
  Subtract2 : Sum  Inputs=+-
  Unit Delay : UnitDelay  SampleTime=-1  HasFrameUpgradeWarning=on
  速度ヘッド : Outport
  wires:
  Constant/1 -> Product/1
  v/1 -> Square/1
  Product/1 -> Divide/2
  Unit Delay/1 -> Subtract2/2
  Square/1 -> Unit Delay/1, Subtract2/1
  Data Store Read1/1 -> Product/2
  Divide/1 -> 速度ヘッド/1
  Subtract2/1 -> Divide/1

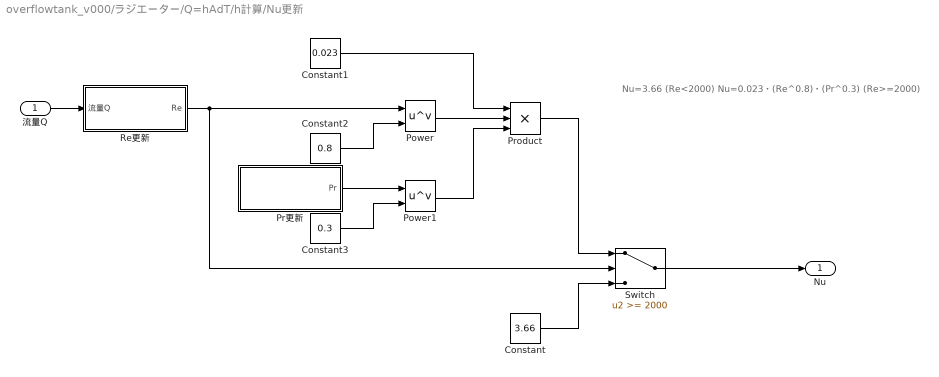
== system overflowtank_v000/ラジエーター/Q=hAdT/h計算/Nu更新 ==
  note: Nu=3.66 (Re<2000)
      | Nu=0.023・(Re^0.8)・(Pr^0.3) (Re>=2000)
  流量Q : Inport
  Constant : Constant  Value=3.66
  Constant1 : Constant  Value=0.023
  Constant2 : Constant  Value=0.8
  Constant3 : Constant  Value=0.3
  Power : Math  Operator=pow  SignedPower=off  SaturateOnIntegerOverflow=on
  Power1 : Math  Operator=pow  SignedPower=off  SaturateOnIntegerOverflow=on
  Product : Product  Inputs=3
  Pr更新 : Subsystem
  Re更新 : Subsystem
  Switch : Switch  Threshold=2000
  Nu : Outport
  wires:
  Constant/1 -> Switch/3
  Switch/1 -> Nu/1
  Re更新/1(Re) -> Switch/2, Power/1
  Constant2/1 -> Power/2
  Pr更新/1(Pr) -> Power1/1
  Constant3/1 -> Power1/2
  Constant1/1 -> Product/1
  Power/1 -> Product/2
  Power1/1 -> Product/3
  Product/1 -> Switch/1
  流量Q/1 -> Re更新/1(流量Q)

== system overflowtank_v000/エンジン/Q=hAdT/h計算 /Nu更新/Pr更新 ==
  note: Pr=μ・Cp/k
  Data Store Read : DataStoreRead  DataStoreName=Cp
  Data Store Read2 : DataStoreRead  DataStoreName=viscosity
  Data Store Read3 : DataStoreRead  DataStoreName=k
  Divide : Product  Inputs=*/
  Product : Product
  Pr : Outport
  wires:
  Data Store Read2/1 -> Product/2
  Data Store Read/1 -> Product/1
  Product/1 -> Divide/1
  Data Store Read3/1 -> Divide/2
  Divide/1 -> Pr/1

== system overflowtank_v000/エンジン/Q=hAdT/h計算 /Nu更新/Re更新 ==
  note: Re=4ρQ/ΠμD
  流量Q : Inport
  Constant : Constant  Value=4
  Constant1 : Constant  Value=pi
  Data Store Read : DataStoreRead  DataStoreName=density
  Data Store Read2 : DataStoreRead  DataStoreName=viscosity
  Data Store Read3 : DataStoreRead  DataStoreName=D
  Divide : Product  Inputs=*/
  Product : Product  Inputs=3
  Product1 : Product  Inputs=3
  Re : Outport
  wires:
  Constant/1 -> Product/1
  Data Store Read/1 -> Product/2
  流量Q/1 -> Product/3
  Product/1 -> Divide/1
  Data Store Read2/1 -> Product1/2
  Constant1/1 -> Product1/1
  Data Store Read3/1 -> Product1/3
  Product1/1 -> Divide/2
  Divide/1 -> Re/1

== system overflowtank_v000/ラジエーター/Q=hAdT/h計算/Nu更新/Pr更新 ==
  note: Pr=μ・Cp/k
  Data Store Read : DataStoreRead  DataStoreName=Cp
  Data Store Read2 : DataStoreRead  DataStoreName=viscosity
  Data Store Read3 : DataStoreRead  DataStoreName=k
  Divide : Product  Inputs=*/
  Product : Product
  Pr : Outport
  wires:
  Data Store Read2/1 -> Product/2
  Data Store Read/1 -> Product/1
  Product/1 -> Divide/1
  Data Store Read3/1 -> Divide/2
  Divide/1 -> Pr/1

== system overflowtank_v000/ラジエーター/Q=hAdT/h計算/Nu更新/Re更新 ==
  note: Re=4ρQ/ΠμD
  流量Q : Inport
  Constant : Constant  Value=4
  Constant1 : Constant  Value=pi
  Data Store Read : DataStoreRead  DataStoreName=density
  Data Store Read2 : DataStoreRead  DataStoreName=viscosity
  Data Store Read3 : DataStoreRead  DataStoreName=D
  Divide : Product  Inputs=*/
  Product : Product  Inputs=3
  Product1 : Product  Inputs=3
  Re : Outport
  wires:
  Constant/1 -> Product/1
  Data Store Read/1 -> Product/2
  流量Q/1 -> Product/3
  Product/1 -> Divide/1
  Data Store Read2/1 -> Product1/2
  Constant1/1 -> Product1/1
  Data Store Read3/1 -> Product1/3
  Product1/1 -> Divide/2
  Divide/1 -> Re/1
